simulink model "autotune1"  (R2018b)
settings: Solver=VariableStepAuto  StartTime=0.0  StopTime=10.0  RelTol=1e-3
libraries: dspvision x3, audiosources x1, dspsnks4 x1
settings Model: Creator=maddiebriere  LastModifiedBy=maddiebriere

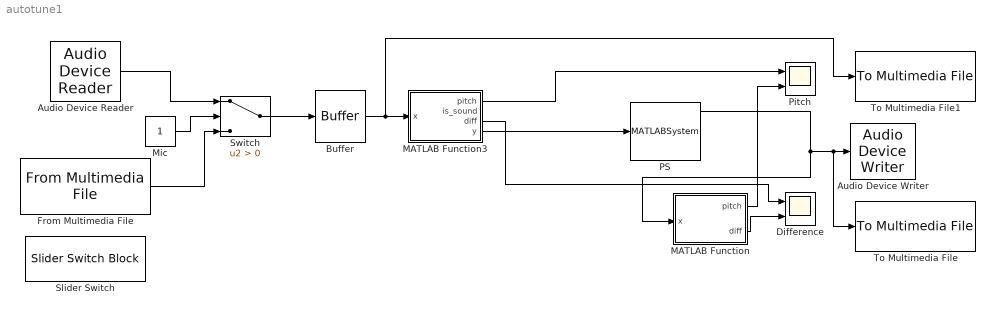
== system autotune1 ==
  Audio Device Reader : audiosources/Audio Device Reader  Driver=CoreAudio  Device=Default  SampleRate=44100  NumChannels=1  SamplesPerFrame=1024  BitDepth=16-bit integer  NumBuffers=10  DefaultInputChannelMapping=on  InputChannelMapping=1:2  OutputNumOverrunSamples=off  OutputDataType=double  DriverIdx=5  DeviceWarnFlag=''
      settings: SourceProductName=Audio Toolbox  SourceProductBaseCode=AU
  Audio Device Writer : dspsnks4/Audio Device Writer  Driver=CoreAudio  Device=Default  InheritSampleRate=on  SampleRate=44100  BitDepth=16-bit integer  BufferSize=4096  NumBuffers=10  DefaultOutputChannelMapping=on  OutputChannelMapping=1:2  OutputNumUnderrunSamples=off  DriverIdx=5  DeviceWarnFlag=''
  Buffer : Buffer  N=4000  OutputFrames=off
  Difference : Scope  NumInputPorts=2
  From Multimedia File : dspvision/From Multimedia File  inputFilename=/Users/maddiebriere/Desktop/Classes/8_Spring 2019/ECE485/ECE485/ECE485Labs/Final/singing44.wav  loop=on  numPlays=inf  outputStreams=Audio only  videoDataType=single  audioDataType=double  inheritSampleTime=on  userDefinedSampleTime=1/30  noAudioOutput=off  isIntensityVideo=off  fourcc=RGB  colorVideoFormat=Separate color signals  outputEOF=off  dataOrg=Column-major  audioFrameSize=1024  computeAudioFrameSize=off  outSamplingMode=Sample based
      settings: SourceProductName=DSP System Toolbox  SourceProductBaseCode=DS
  MATLAB Function : MATLAB Function  TreatAsAtomicUnit=on
  MATLAB Function3 : MATLAB Function  TreatAsAtomicUnit=on
  Mic : Constant
  PS : MATLABSystem  System=PitchShifter  PitchShift=0  Overlap=0.01  SimulateUsing=Code generation
      mask Type: PitchShifter
      mask Display:
      | disp('PitchShifter');
      | port_label('input',1,'u');
      | port_label('output',1,'y');
      | port_label('output',2,'delays');
      | port_label('output',3,'gains');
  Pitch : Scope  NumInputPorts=2
  Slider Switch : SliderSwitchBlock
      settings: Values={{'Off', 'On'}, [0 1]}
  Switch : Switch  Criteria=u2 > Threshold
  To Multimedia File : dspvision/To Multimedia File  outputFilename=output.wav  streamSelection=Audio only  videoCompressor=None (uncompressed)  audioCompressor=None (uncompressed)  imagePorts=Separate color signals  fileType=WAV  audioDatatype=16-bit integer  fourcc=RGB  videoQuality=75  mj2000CompFactor=10
      settings: SourceProductName=DSP System Toolbox  SourceProductBaseCode=DS
  To Multimedia File1 : dspvision/To Multimedia File  outputFilename=input.wav  streamSelection=Audio only  videoCompressor=None (uncompressed)  audioCompressor=None (uncompressed)  imagePorts=Separate color signals  fileType=WAV  audioDatatype=16-bit integer  fourcc=RGB  videoQuality=75  mj2000CompFactor=10
      settings: SourceProductName=DSP System Toolbox  SourceProductBaseCode=DS
  wires:
  PS/1 -> To Multimedia File/1, Audio Device Writer/1, MATLAB Function/1(x)
  MATLAB Function/2(diff) -> Difference/2
  MATLAB Function3/3(diff) -> Difference/1
  Buffer/1 -> To Multimedia File1/1, MATLAB Function3/1(x)
  Audio Device Reader/1 -> Switch/1
  From Multimedia File/1 -> Switch/3
  Switch/1 -> Buffer/1
  Mic/1 -> Switch/2
  MATLAB Function3/1(pitch) -> Pitch/1
  MATLAB Function3/4(y) -> PS/1
  MATLAB Function/1(pitch) -> Pitch/2

== matlab function autotune1/MATLAB Function ==
  data: pitch output; x input; diff output
function [pitch, diff] = fcn(x)
[pitch, ~, diff] = autotune_fcn(x);
end

== matlab function autotune1/MATLAB Function3 ==
  data: x input; pitch output; is_sound output; diff output; y output
function [pitch, is_sound, diff, y] = fcn(x)
[pitch, is_sound, diff] = autotune_fcn(x);
coder.extrinsic('set_param')
coder.extrinsic('num2str')
set_param('autotune/PS', 'PitchShift', num2str(diff));
y = x;
end
